simulink subsystem "linear_plant"  (R2022b)
settings: Solver=VariableStepAuto  StartTime=0.0  StopTime=10.0  RelTol=1e-3
undefined symbols (not defined in the file or in its folder): param
settings Model: Creator=Alex Zhen  LastModifiedBy=Alex Zhen

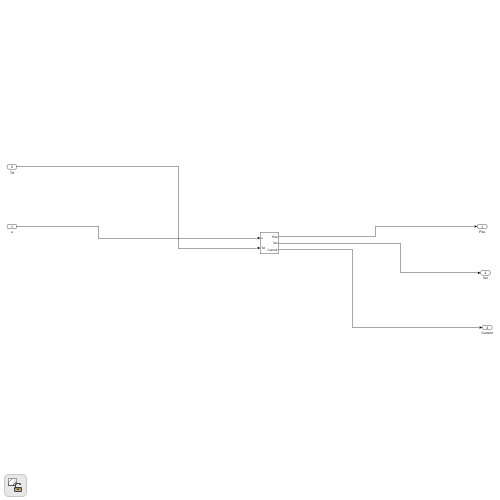
[thumbnail: Simulink's stored preview of the top-level diagram]
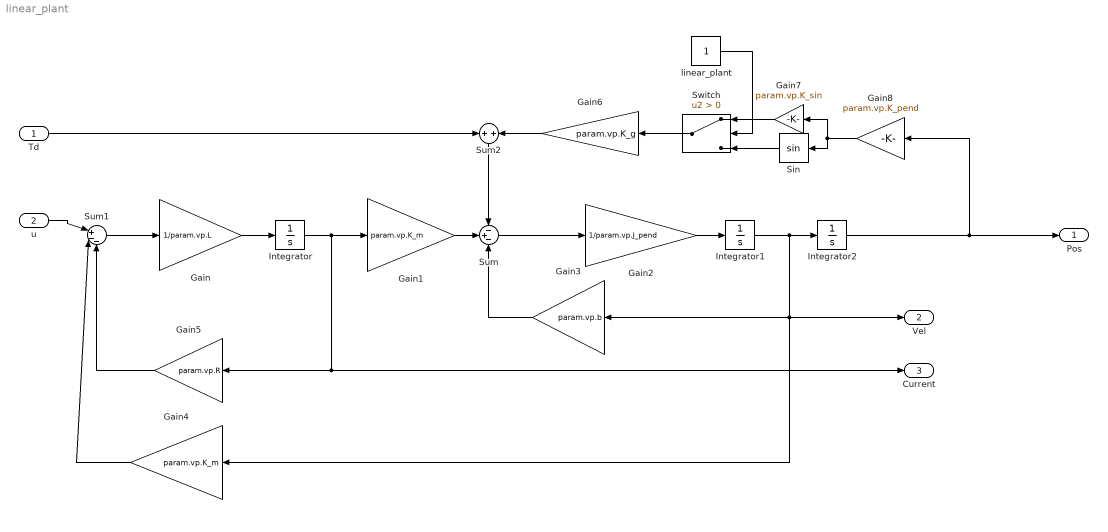
== system linear_plant ==
  Td : Inport
  u : Inport  Port=2
  Gain : Gain  Gain=1/param.vp.L
  Gain1 : Gain  Gain=param.vp.K_m
  Gain2 : Gain  Gain=1/param.vp.J_pend
  Gain3 : Gain  Gain=param.vp.b
  Gain4 : Gain  Gain=param.vp.K_m
  Gain5 : Gain  Gain=param.vp.R
  Gain6 : Gain  Gain=param.vp.K_g
  Gain7 : Gain  Gain=param.vp.K_sin
  Gain8 : Gain  Gain=param.vp.K_pend
  Integrator : Integrator
  Integrator1 : Integrator
  Integrator2 : Integrator
  Sin : Trigonometry
  Sum : Sum  Inputs=-+-
  Sum1 : Sum  Inputs=|+--
  Sum2 : Sum
  Switch : Switch  Criteria=u2 > Threshold  SaturateOnIntegerOverflow=off  InputSameDT=off
  linear_plant : Constant
  Pos : Outport
  Vel : Outport  Port=2
  Current : Outport  Port=3
  wires:
  Td/1 -> Sum2/1
  u/1 -> Sum1/1
  Gain5/1 -> Sum1/3
  Gain1/1 -> Sum/2
  Gain2/1 -> Integrator1/1
  Sum/1 -> Gain2/1
  Integrator/1 -> Gain1/1, Current/1, Gain5/1
  Integrator2/1 -> Pos/1, Gain8/1
  Sum1/1 -> Gain/1
  Gain/1 -> Integrator/1
  Gain4/1 -> Sum1/2
  Integrator1/1 -> Vel/1, Gain3/1, Gain4/1, Integrator2/1
  Gain3/1 -> Sum/3
  Sum2/1 -> Sum/1
  Gain6/1 -> Sum2/2
  Gain7/1 -> Switch/1
  Switch/1 -> Gain6/1
  Sin/1 -> Switch/3
  Gain8/1 -> Sin/1, Gain7/1
  linear_plant/1 -> Switch/2
